simulink model "Multiplier"  (R2017b)
settings: Solver=ode45  StartTime=0.0  StopTime=10.0  RelTol=1e-3  EnableMultiTasking=on
libraries: hdlsllib x17
(part 2 of 3)

== system Multiplier/8-bit_Multiplier/Multiplier/Multiplier Building Block54 ==
  Cin : Inport
  X : Inport  Port=2
  Y : Inport  Port=3
  Sum in : Inport  Port=4
  AND : Logic  IconShape=distinctive  AllPortsSameDT=off  OutDataTypeStr=boolean
  Full Adder : Subsystem
  Sum Out : Outport
  C Out : Outport  Port=2
  wires:
  Cin/1 -> Full Adder/3(Z)
  Sum in/1 -> Full Adder/1(X)
  AND/1 -> Full Adder/2(Y)
  Full Adder/1(S) -> Sum Out/1
  Y/1 -> AND/2
  X/1 -> AND/1
  Full Adder/2(C) -> C Out/1

== system Multiplier/8-bit_Multiplier/Multiplier/Multiplier Building Block55 ==
  Cin : Inport
  X : Inport  Port=2
  Y : Inport  Port=3
  Sum in : Inport  Port=4
  AND : Logic  IconShape=distinctive  AllPortsSameDT=off  OutDataTypeStr=boolean
  Full Adder : Subsystem
  Sum Out : Outport
  C Out : Outport  Port=2
  wires:
  Cin/1 -> Full Adder/3(Z)
  Sum in/1 -> Full Adder/1(X)
  AND/1 -> Full Adder/2(Y)
  Full Adder/1(S) -> Sum Out/1
  Y/1 -> AND/2
  X/1 -> AND/1
  Full Adder/2(C) -> C Out/1

== system Multiplier/8-bit_Multiplier/Multiplier/Multiplier Building Block56 ==
  Cin : Inport
  X : Inport  Port=2
  Y : Inport  Port=3
  Sum in : Inport  Port=4
  AND : Logic  IconShape=distinctive  AllPortsSameDT=off  OutDataTypeStr=boolean
  Full Adder : Subsystem
  Sum Out : Outport
  C Out : Outport  Port=2
  wires:
  Cin/1 -> Full Adder/3(Z)
  Sum in/1 -> Full Adder/1(X)
  AND/1 -> Full Adder/2(Y)
  Full Adder/1(S) -> Sum Out/1
  Y/1 -> AND/2
  X/1 -> AND/1
  Full Adder/2(C) -> C Out/1

== system Multiplier/8-bit_Multiplier/Multiplier/Multiplier Building Block57 ==
  Cin : Inport
  X : Inport  Port=2
  Y : Inport  Port=3
  Sum in : Inport  Port=4
  AND : Logic  IconShape=distinctive  AllPortsSameDT=off  OutDataTypeStr=boolean
  Full Adder : Subsystem
  Sum Out : Outport
  C Out : Outport  Port=2
  wires:
  Cin/1 -> Full Adder/3(Z)
  Sum in/1 -> Full Adder/1(X)
  AND/1 -> Full Adder/2(Y)
  Full Adder/1(S) -> Sum Out/1
  Y/1 -> AND/2
  X/1 -> AND/1
  Full Adder/2(C) -> C Out/1

== system Multiplier/8-bit_Multiplier/Multiplier/Multiplier Building Block58 ==
  Cin : Inport
  X : Inport  Port=2
  Y : Inport  Port=3
  Sum in : Inport  Port=4
  AND : Logic  IconShape=distinctive  AllPortsSameDT=off  OutDataTypeStr=boolean
  Full Adder : Subsystem
  Sum Out : Outport
  C Out : Outport  Port=2
  wires:
  Cin/1 -> Full Adder/3(Z)
  Sum in/1 -> Full Adder/1(X)
  AND/1 -> Full Adder/2(Y)
  Full Adder/1(S) -> Sum Out/1
  Y/1 -> AND/2
  X/1 -> AND/1
  Full Adder/2(C) -> C Out/1

== system Multiplier/8-bit_Multiplier/Multiplier/Multiplier Building Block59 ==
  Cin : Inport
  X : Inport  Port=2
  Y : Inport  Port=3
  Sum in : Inport  Port=4
  AND : Logic  IconShape=distinctive  AllPortsSameDT=off  OutDataTypeStr=boolean
  Full Adder : Subsystem
  Sum Out : Outport
  C Out : Outport  Port=2
  wires:
  Cin/1 -> Full Adder/3(Z)
  Sum in/1 -> Full Adder/1(X)
  AND/1 -> Full Adder/2(Y)
  Full Adder/1(S) -> Sum Out/1
  Y/1 -> AND/2
  X/1 -> AND/1
  Full Adder/2(C) -> C Out/1

== system Multiplier/8-bit_Multiplier/Multiplier/Multiplier Building Block6 ==
  Cin : Inport
  X : Inport  Port=2
  Y : Inport  Port=3
  Sum in : Inport  Port=4
  AND : Logic  IconShape=distinctive  AllPortsSameDT=off  OutDataTypeStr=boolean
  Full Adder : Subsystem
  Sum Out : Outport
  C Out : Outport  Port=2
  wires:
  Cin/1 -> Full Adder/3(Z)
  Sum in/1 -> Full Adder/1(X)
  AND/1 -> Full Adder/2(Y)
  Full Adder/1(S) -> Sum Out/1
  Y/1 -> AND/2
  X/1 -> AND/1
  Full Adder/2(C) -> C Out/1

== system Multiplier/8-bit_Multiplier/Multiplier/Multiplier Building Block60 ==
  Cin : Inport
  X : Inport  Port=2
  Y : Inport  Port=3
  Sum in : Inport  Port=4
  AND : Logic  IconShape=distinctive  AllPortsSameDT=off  OutDataTypeStr=boolean
  Full Adder : Subsystem
  Sum Out : Outport
  C Out : Outport  Port=2
  wires:
  Cin/1 -> Full Adder/3(Z)
  Sum in/1 -> Full Adder/1(X)
  AND/1 -> Full Adder/2(Y)
  Full Adder/1(S) -> Sum Out/1
  Y/1 -> AND/2
  X/1 -> AND/1
  Full Adder/2(C) -> C Out/1

== system Multiplier/8-bit_Multiplier/Multiplier/Multiplier Building Block61 ==
  Cin : Inport
  X : Inport  Port=2
  Y : Inport  Port=3
  Sum in : Inport  Port=4
  AND : Logic  IconShape=distinctive  AllPortsSameDT=off  OutDataTypeStr=boolean
  Full Adder : Subsystem
  Sum Out : Outport
  C Out : Outport  Port=2
  wires:
  Cin/1 -> Full Adder/3(Z)
  Sum in/1 -> Full Adder/1(X)
  AND/1 -> Full Adder/2(Y)
  Full Adder/1(S) -> Sum Out/1
  Y/1 -> AND/2
  X/1 -> AND/1
  Full Adder/2(C) -> C Out/1

== system Multiplier/8-bit_Multiplier/Multiplier/Multiplier Building Block62 ==
  Cin : Inport
  X : Inport  Port=2
  Y : Inport  Port=3
  Sum in : Inport  Port=4
  AND : Logic  IconShape=distinctive  AllPortsSameDT=off  OutDataTypeStr=boolean
  Full Adder : Subsystem
  Sum Out : Outport
  C Out : Outport  Port=2
  wires:
  Cin/1 -> Full Adder/3(Z)
  Sum in/1 -> Full Adder/1(X)
  AND/1 -> Full Adder/2(Y)
  Full Adder/1(S) -> Sum Out/1
  Y/1 -> AND/2
  X/1 -> AND/1
  Full Adder/2(C) -> C Out/1

== system Multiplier/8-bit_Multiplier/Multiplier/Multiplier Building Block63 ==
  Cin : Inport
  X : Inport  Port=2
  Y : Inport  Port=3
  Sum in : Inport  Port=4
  AND : Logic  IconShape=distinctive  AllPortsSameDT=off  OutDataTypeStr=boolean
  Full Adder : Subsystem
  Sum Out : Outport
  C Out : Outport  Port=2
  wires:
  Cin/1 -> Full Adder/3(Z)
  Sum in/1 -> Full Adder/1(X)
  AND/1 -> Full Adder/2(Y)
  Full Adder/1(S) -> Sum Out/1
  Y/1 -> AND/2
  X/1 -> AND/1
  Full Adder/2(C) -> C Out/1

== system Multiplier/8-bit_Multiplier/Multiplier/Multiplier Building Block7 ==
  Cin : Inport
  X : Inport  Port=2
  Y : Inport  Port=3
  Sum in : Inport  Port=4
  AND : Logic  IconShape=distinctive  AllPortsSameDT=off  OutDataTypeStr=boolean
  Full Adder : Subsystem
  Sum Out : Outport
  C Out : Outport  Port=2
  wires:
  Cin/1 -> Full Adder/3(Z)
  Sum in/1 -> Full Adder/1(X)
  AND/1 -> Full Adder/2(Y)
  Full Adder/1(S) -> Sum Out/1
  Y/1 -> AND/2
  X/1 -> AND/1
  Full Adder/2(C) -> C Out/1

== system Multiplier/8-bit_Multiplier/Multiplier/Multiplier Building Block8 ==
  Cin : Inport
  X : Inport  Port=2
  Y : Inport  Port=3
  Sum in : Inport  Port=4
  AND : Logic  IconShape=distinctive  AllPortsSameDT=off  OutDataTypeStr=boolean
  Full Adder : Subsystem
  Sum Out : Outport
  C Out : Outport  Port=2
  wires:
  Cin/1 -> Full Adder/3(Z)
  Sum in/1 -> Full Adder/1(X)
  AND/1 -> Full Adder/2(Y)
  Full Adder/1(S) -> Sum Out/1
  Y/1 -> AND/2
  X/1 -> AND/1
  Full Adder/2(C) -> C Out/1

== system Multiplier/8-bit_Multiplier/Multiplier/Multiplier Building Block9 ==
  Cin : Inport
  X : Inport  Port=2
  Y : Inport  Port=3
  Sum in : Inport  Port=4
  AND : Logic  IconShape=distinctive  AllPortsSameDT=off  OutDataTypeStr=boolean
  Full Adder : Subsystem
  Sum Out : Outport
  C Out : Outport  Port=2
  wires:
  Cin/1 -> Full Adder/3(Z)
  Sum in/1 -> Full Adder/1(X)
  AND/1 -> Full Adder/2(Y)
  Full Adder/1(S) -> Sum Out/1
  Y/1 -> AND/2
  X/1 -> AND/1
  Full Adder/2(C) -> C Out/1

== system Multiplier/8-bit_Multiplier/Multiplier/Multiplier Building Block/Full Adder ==
  X : Inport
  Y : Inport  Port=2
  Z : Inport  Port=3
  Half Adder : Subsystem
  Half Adder1 : Subsystem
  OR : Logic  Operator=OR  IconShape=distinctive  AllPortsSameDT=off  OutDataTypeStr=boolean
  S : Outport
  C : Outport  Port=2
  wires:
  Half Adder1/1(Sum) -> S/1
  Half Adder/1(Sum) -> Half Adder1/1(A)
  Half Adder/2(Carry) -> OR/2
  X/1 -> Half Adder/1(A)
  Z/1 -> Half Adder1/2(B)
  OR/1 -> C/1
  Y/1 -> Half Adder/2(B)
  Half Adder1/2(Carry) -> OR/1

== system Multiplier/8-bit_Multiplier/Multiplier/Multiplier Building Block1/Full Adder ==
  X : Inport
  Y : Inport  Port=2
  Z : Inport  Port=3
  Half Adder : Subsystem
  Half Adder1 : Subsystem
  OR : Logic  Operator=OR  IconShape=distinctive  AllPortsSameDT=off  OutDataTypeStr=boolean
  S : Outport
  C : Outport  Port=2
  wires:
  Half Adder1/1(Sum) -> S/1
  Half Adder/1(Sum) -> Half Adder1/1(A)
  Half Adder/2(Carry) -> OR/2
  X/1 -> Half Adder/1(A)
  Z/1 -> Half Adder1/2(B)
  OR/1 -> C/1
  Y/1 -> Half Adder/2(B)
  Half Adder1/2(Carry) -> OR/1

== system Multiplier/8-bit_Multiplier/Multiplier/Multiplier Building Block10/Full Adder ==
  X : Inport
  Y : Inport  Port=2
  Z : Inport  Port=3
  Half Adder : Subsystem
  Half Adder1 : Subsystem
  OR : Logic  Operator=OR  IconShape=distinctive  AllPortsSameDT=off  OutDataTypeStr=boolean
  S : Outport
  C : Outport  Port=2
  wires:
  Half Adder1/1(Sum) -> S/1
  Half Adder/1(Sum) -> Half Adder1/1(A)
  Half Adder/2(Carry) -> OR/2
  X/1 -> Half Adder/1(A)
  Z/1 -> Half Adder1/2(B)
  OR/1 -> C/1
  Y/1 -> Half Adder/2(B)
  Half Adder1/2(Carry) -> OR/1

== system Multiplier/8-bit_Multiplier/Multiplier/Multiplier Building Block11/Full Adder ==
  X : Inport
  Y : Inport  Port=2
  Z : Inport  Port=3
  Half Adder : Subsystem
  Half Adder1 : Subsystem
  OR : Logic  Operator=OR  IconShape=distinctive  AllPortsSameDT=off  OutDataTypeStr=boolean
  S : Outport
  C : Outport  Port=2
  wires:
  Half Adder1/1(Sum) -> S/1
  Half Adder/1(Sum) -> Half Adder1/1(A)
  Half Adder/2(Carry) -> OR/2
  X/1 -> Half Adder/1(A)
  Z/1 -> Half Adder1/2(B)
  OR/1 -> C/1
  Y/1 -> Half Adder/2(B)
  Half Adder1/2(Carry) -> OR/1

== system Multiplier/8-bit_Multiplier/Multiplier/Multiplier Building Block12/Full Adder ==
  X : Inport
  Y : Inport  Port=2
  Z : Inport  Port=3
  Half Adder : Subsystem
  Half Adder1 : Subsystem
  OR : Logic  Operator=OR  IconShape=distinctive  AllPortsSameDT=off  OutDataTypeStr=boolean
  S : Outport
  C : Outport  Port=2
  wires:
  Half Adder1/1(Sum) -> S/1
  Half Adder/1(Sum) -> Half Adder1/1(A)
  Half Adder/2(Carry) -> OR/2
  X/1 -> Half Adder/1(A)
  Z/1 -> Half Adder1/2(B)
  OR/1 -> C/1
  Y/1 -> Half Adder/2(B)
  Half Adder1/2(Carry) -> OR/1

== system Multiplier/8-bit_Multiplier/Multiplier/Multiplier Building Block13/Full Adder ==
  X : Inport
  Y : Inport  Port=2
  Z : Inport  Port=3
  Half Adder : Subsystem
  Half Adder1 : Subsystem
  OR : Logic  Operator=OR  IconShape=distinctive  AllPortsSameDT=off  OutDataTypeStr=boolean
  S : Outport
  C : Outport  Port=2
  wires:
  Half Adder1/1(Sum) -> S/1
  Half Adder/1(Sum) -> Half Adder1/1(A)
  Half Adder/2(Carry) -> OR/2
  X/1 -> Half Adder/1(A)
  Z/1 -> Half Adder1/2(B)
  OR/1 -> C/1
  Y/1 -> Half Adder/2(B)
  Half Adder1/2(Carry) -> OR/1

== system Multiplier/8-bit_Multiplier/Multiplier/Multiplier Building Block14/Full Adder ==
  X : Inport
  Y : Inport  Port=2
  Z : Inport  Port=3
  Half Adder : Subsystem
  Half Adder1 : Subsystem
  OR : Logic  Operator=OR  IconShape=distinctive  AllPortsSameDT=off  OutDataTypeStr=boolean
  S : Outport
  C : Outport  Port=2
  wires:
  Half Adder1/1(Sum) -> S/1
  Half Adder/1(Sum) -> Half Adder1/1(A)
  Half Adder/2(Carry) -> OR/2
  X/1 -> Half Adder/1(A)
  Z/1 -> Half Adder1/2(B)
  OR/1 -> C/1
  Y/1 -> Half Adder/2(B)
  Half Adder1/2(Carry) -> OR/1

== system Multiplier/8-bit_Multiplier/Multiplier/Multiplier Building Block15/Full Adder ==
  X : Inport
  Y : Inport  Port=2
  Z : Inport  Port=3
  Half Adder : Subsystem
  Half Adder1 : Subsystem
  OR : Logic  Operator=OR  IconShape=distinctive  AllPortsSameDT=off  OutDataTypeStr=boolean
  S : Outport
  C : Outport  Port=2
  wires:
  Half Adder1/1(Sum) -> S/1
  Half Adder/1(Sum) -> Half Adder1/1(A)
  Half Adder/2(Carry) -> OR/2
  X/1 -> Half Adder/1(A)
  Z/1 -> Half Adder1/2(B)
  OR/1 -> C/1
  Y/1 -> Half Adder/2(B)
  Half Adder1/2(Carry) -> OR/1

== system Multiplier/8-bit_Multiplier/Multiplier/Multiplier Building Block16/Full Adder ==
  X : Inport
  Y : Inport  Port=2
  Z : Inport  Port=3
  Half Adder : Subsystem
  Half Adder1 : Subsystem
  OR : Logic  Operator=OR  IconShape=distinctive  AllPortsSameDT=off  OutDataTypeStr=boolean
  S : Outport
  C : Outport  Port=2
  wires:
  Half Adder1/1(Sum) -> S/1
  Half Adder/1(Sum) -> Half Adder1/1(A)
  Half Adder/2(Carry) -> OR/2
  X/1 -> Half Adder/1(A)
  Z/1 -> Half Adder1/2(B)
  OR/1 -> C/1
  Y/1 -> Half Adder/2(B)
  Half Adder1/2(Carry) -> OR/1

== system Multiplier/8-bit_Multiplier/Multiplier/Multiplier Building Block17/Full Adder ==
  X : Inport
  Y : Inport  Port=2
  Z : Inport  Port=3
  Half Adder : Subsystem
  Half Adder1 : Subsystem
  OR : Logic  Operator=OR  IconShape=distinctive  AllPortsSameDT=off  OutDataTypeStr=boolean
  S : Outport
  C : Outport  Port=2
  wires:
  Half Adder1/1(Sum) -> S/1
  Half Adder/1(Sum) -> Half Adder1/1(A)
  Half Adder/2(Carry) -> OR/2
  X/1 -> Half Adder/1(A)
  Z/1 -> Half Adder1/2(B)
  OR/1 -> C/1
  Y/1 -> Half Adder/2(B)
  Half Adder1/2(Carry) -> OR/1

== system Multiplier/8-bit_Multiplier/Multiplier/Multiplier Building Block18/Full Adder ==
  X : Inport
  Y : Inport  Port=2
  Z : Inport  Port=3
  Half Adder : Subsystem
  Half Adder1 : Subsystem
  OR : Logic  Operator=OR  IconShape=distinctive  AllPortsSameDT=off  OutDataTypeStr=boolean
  S : Outport
  C : Outport  Port=2
  wires:
  Half Adder1/1(Sum) -> S/1
  Half Adder/1(Sum) -> Half Adder1/1(A)
  Half Adder/2(Carry) -> OR/2
  X/1 -> Half Adder/1(A)
  Z/1 -> Half Adder1/2(B)
  OR/1 -> C/1
  Y/1 -> Half Adder/2(B)
  Half Adder1/2(Carry) -> OR/1

== system Multiplier/8-bit_Multiplier/Multiplier/Multiplier Building Block19/Full Adder ==
  X : Inport
  Y : Inport  Port=2
  Z : Inport  Port=3
  Half Adder : Subsystem
  Half Adder1 : Subsystem
  OR : Logic  Operator=OR  IconShape=distinctive  AllPortsSameDT=off  OutDataTypeStr=boolean
  S : Outport
  C : Outport  Port=2
  wires:
  Half Adder1/1(Sum) -> S/1
  Half Adder/1(Sum) -> Half Adder1/1(A)
  Half Adder/2(Carry) -> OR/2
  X/1 -> Half Adder/1(A)
  Z/1 -> Half Adder1/2(B)
  OR/1 -> C/1
  Y/1 -> Half Adder/2(B)
  Half Adder1/2(Carry) -> OR/1

== system Multiplier/8-bit_Multiplier/Multiplier/Multiplier Building Block2/Full Adder ==
  X : Inport
  Y : Inport  Port=2
  Z : Inport  Port=3
  Half Adder : Subsystem
  Half Adder1 : Subsystem
  OR : Logic  Operator=OR  IconShape=distinctive  AllPortsSameDT=off  OutDataTypeStr=boolean
  S : Outport
  C : Outport  Port=2
  wires:
  Half Adder1/1(Sum) -> S/1
  Half Adder/1(Sum) -> Half Adder1/1(A)
  Half Adder/2(Carry) -> OR/2
  X/1 -> Half Adder/1(A)
  Z/1 -> Half Adder1/2(B)
  OR/1 -> C/1
  Y/1 -> Half Adder/2(B)
  Half Adder1/2(Carry) -> OR/1

== system Multiplier/8-bit_Multiplier/Multiplier/Multiplier Building Block20/Full Adder ==
  X : Inport
  Y : Inport  Port=2
  Z : Inport  Port=3
  Half Adder : Subsystem
  Half Adder1 : Subsystem
  OR : Logic  Operator=OR  IconShape=distinctive  AllPortsSameDT=off  OutDataTypeStr=boolean
  S : Outport
  C : Outport  Port=2
  wires:
  Half Adder1/1(Sum) -> S/1
  Half Adder/1(Sum) -> Half Adder1/1(A)
  Half Adder/2(Carry) -> OR/2
  X/1 -> Half Adder/1(A)
  Z/1 -> Half Adder1/2(B)
  OR/1 -> C/1
  Y/1 -> Half Adder/2(B)
  Half Adder1/2(Carry) -> OR/1

== system Multiplier/8-bit_Multiplier/Multiplier/Multiplier Building Block21/Full Adder ==
  X : Inport
  Y : Inport  Port=2
  Z : Inport  Port=3
  Half Adder : Subsystem
  Half Adder1 : Subsystem
  OR : Logic  Operator=OR  IconShape=distinctive  AllPortsSameDT=off  OutDataTypeStr=boolean
  S : Outport
  C : Outport  Port=2
  wires:
  Half Adder1/1(Sum) -> S/1
  Half Adder/1(Sum) -> Half Adder1/1(A)
  Half Adder/2(Carry) -> OR/2
  X/1 -> Half Adder/1(A)
  Z/1 -> Half Adder1/2(B)
  OR/1 -> C/1
  Y/1 -> Half Adder/2(B)
  Half Adder1/2(Carry) -> OR/1

== system Multiplier/8-bit_Multiplier/Multiplier/Multiplier Building Block22/Full Adder ==
  X : Inport
  Y : Inport  Port=2
  Z : Inport  Port=3
  Half Adder : Subsystem
  Half Adder1 : Subsystem
  OR : Logic  Operator=OR  IconShape=distinctive  AllPortsSameDT=off  OutDataTypeStr=boolean
  S : Outport
  C : Outport  Port=2
  wires:
  Half Adder1/1(Sum) -> S/1
  Half Adder/1(Sum) -> Half Adder1/1(A)
  Half Adder/2(Carry) -> OR/2
  X/1 -> Half Adder/1(A)
  Z/1 -> Half Adder1/2(B)
  OR/1 -> C/1
  Y/1 -> Half Adder/2(B)
  Half Adder1/2(Carry) -> OR/1

== system Multiplier/8-bit_Multiplier/Multiplier/Multiplier Building Block23/Full Adder ==
  X : Inport
  Y : Inport  Port=2
  Z : Inport  Port=3
  Half Adder : Subsystem
  Half Adder1 : Subsystem
  OR : Logic  Operator=OR  IconShape=distinctive  AllPortsSameDT=off  OutDataTypeStr=boolean
  S : Outport
  C : Outport  Port=2
  wires:
  Half Adder1/1(Sum) -> S/1
  Half Adder/1(Sum) -> Half Adder1/1(A)
  Half Adder/2(Carry) -> OR/2
  X/1 -> Half Adder/1(A)
  Z/1 -> Half Adder1/2(B)
  OR/1 -> C/1
  Y/1 -> Half Adder/2(B)
  Half Adder1/2(Carry) -> OR/1

== system Multiplier/8-bit_Multiplier/Multiplier/Multiplier Building Block24/Full Adder ==
  X : Inport
  Y : Inport  Port=2
  Z : Inport  Port=3
  Half Adder : Subsystem
  Half Adder1 : Subsystem
  OR : Logic  Operator=OR  IconShape=distinctive  AllPortsSameDT=off  OutDataTypeStr=boolean
  S : Outport
  C : Outport  Port=2
  wires:
  Half Adder1/1(Sum) -> S/1
  Half Adder/1(Sum) -> Half Adder1/1(A)
  Half Adder/2(Carry) -> OR/2
  X/1 -> Half Adder/1(A)
  Z/1 -> Half Adder1/2(B)
  OR/1 -> C/1
  Y/1 -> Half Adder/2(B)
  Half Adder1/2(Carry) -> OR/1

== system Multiplier/8-bit_Multiplier/Multiplier/Multiplier Building Block25/Full Adder ==
  X : Inport
  Y : Inport  Port=2
  Z : Inport  Port=3
  Half Adder : Subsystem
  Half Adder1 : Subsystem
  OR : Logic  Operator=OR  IconShape=distinctive  AllPortsSameDT=off  OutDataTypeStr=boolean
  S : Outport
  C : Outport  Port=2
  wires:
  Half Adder1/1(Sum) -> S/1
  Half Adder/1(Sum) -> Half Adder1/1(A)
  Half Adder/2(Carry) -> OR/2
  X/1 -> Half Adder/1(A)
  Z/1 -> Half Adder1/2(B)
  OR/1 -> C/1
  Y/1 -> Half Adder/2(B)
  Half Adder1/2(Carry) -> OR/1

== system Multiplier/8-bit_Multiplier/Multiplier/Multiplier Building Block26/Full Adder ==
  X : Inport
  Y : Inport  Port=2
  Z : Inport  Port=3
  Half Adder : Subsystem
  Half Adder1 : Subsystem
  OR : Logic  Operator=OR  IconShape=distinctive  AllPortsSameDT=off  OutDataTypeStr=boolean
  S : Outport
  C : Outport  Port=2
  wires:
  Half Adder1/1(Sum) -> S/1
  Half Adder/1(Sum) -> Half Adder1/1(A)
  Half Adder/2(Carry) -> OR/2
  X/1 -> Half Adder/1(A)
  Z/1 -> Half Adder1/2(B)
  OR/1 -> C/1
  Y/1 -> Half Adder/2(B)
  Half Adder1/2(Carry) -> OR/1

== system Multiplier/8-bit_Multiplier/Multiplier/Multiplier Building Block27/Full Adder ==
  X : Inport
  Y : Inport  Port=2
  Z : Inport  Port=3
  Half Adder : Subsystem
  Half Adder1 : Subsystem
  OR : Logic  Operator=OR  IconShape=distinctive  AllPortsSameDT=off  OutDataTypeStr=boolean
  S : Outport
  C : Outport  Port=2
  wires:
  Half Adder1/1(Sum) -> S/1
  Half Adder/1(Sum) -> Half Adder1/1(A)
  Half Adder/2(Carry) -> OR/2
  X/1 -> Half Adder/1(A)
  Z/1 -> Half Adder1/2(B)
  OR/1 -> C/1
  Y/1 -> Half Adder/2(B)
  Half Adder1/2(Carry) -> OR/1

== system Multiplier/8-bit_Multiplier/Multiplier/Multiplier Building Block28/Full Adder ==
  X : Inport
  Y : Inport  Port=2
  Z : Inport  Port=3
  Half Adder : Subsystem
  Half Adder1 : Subsystem
  OR : Logic  Operator=OR  IconShape=distinctive  AllPortsSameDT=off  OutDataTypeStr=boolean
  S : Outport
  C : Outport  Port=2
  wires:
  Half Adder1/1(Sum) -> S/1
  Half Adder/1(Sum) -> Half Adder1/1(A)
  Half Adder/2(Carry) -> OR/2
  X/1 -> Half Adder/1(A)
  Z/1 -> Half Adder1/2(B)
  OR/1 -> C/1
  Y/1 -> Half Adder/2(B)
  Half Adder1/2(Carry) -> OR/1

== system Multiplier/8-bit_Multiplier/Multiplier/Multiplier Building Block29/Full Adder ==
  X : Inport
  Y : Inport  Port=2
  Z : Inport  Port=3
  Half Adder : Subsystem
  Half Adder1 : Subsystem
  OR : Logic  Operator=OR  IconShape=distinctive  AllPortsSameDT=off  OutDataTypeStr=boolean
  S : Outport
  C : Outport  Port=2
  wires:
  Half Adder1/1(Sum) -> S/1
  Half Adder/1(Sum) -> Half Adder1/1(A)
  Half Adder/2(Carry) -> OR/2
  X/1 -> Half Adder/1(A)
  Z/1 -> Half Adder1/2(B)
  OR/1 -> C/1
  Y/1 -> Half Adder/2(B)
  Half Adder1/2(Carry) -> OR/1

== system Multiplier/8-bit_Multiplier/Multiplier/Multiplier Building Block3/Full Adder ==
  X : Inport
  Y : Inport  Port=2
  Z : Inport  Port=3
  Half Adder : Subsystem
  Half Adder1 : Subsystem
  OR : Logic  Operator=OR  IconShape=distinctive  AllPortsSameDT=off  OutDataTypeStr=boolean
  S : Outport
  C : Outport  Port=2
  wires:
  Half Adder1/1(Sum) -> S/1
  Half Adder/1(Sum) -> Half Adder1/1(A)
  Half Adder/2(Carry) -> OR/2
  X/1 -> Half Adder/1(A)
  Z/1 -> Half Adder1/2(B)
  OR/1 -> C/1
  Y/1 -> Half Adder/2(B)
  Half Adder1/2(Carry) -> OR/1

== system Multiplier/8-bit_Multiplier/Multiplier/Multiplier Building Block30/Full Adder ==
  X : Inport
  Y : Inport  Port=2
  Z : Inport  Port=3
  Half Adder : Subsystem
  Half Adder1 : Subsystem
  OR : Logic  Operator=OR  IconShape=distinctive  AllPortsSameDT=off  OutDataTypeStr=boolean
  S : Outport
  C : Outport  Port=2
  wires:
  Half Adder1/1(Sum) -> S/1
  Half Adder/1(Sum) -> Half Adder1/1(A)
  Half Adder/2(Carry) -> OR/2
  X/1 -> Half Adder/1(A)
  Z/1 -> Half Adder1/2(B)
  OR/1 -> C/1
  Y/1 -> Half Adder/2(B)
  Half Adder1/2(Carry) -> OR/1

== system Multiplier/8-bit_Multiplier/Multiplier/Multiplier Building Block31/Full Adder ==
  X : Inport
  Y : Inport  Port=2
  Z : Inport  Port=3
  Half Adder : Subsystem
  Half Adder1 : Subsystem
  OR : Logic  Operator=OR  IconShape=distinctive  AllPortsSameDT=off  OutDataTypeStr=boolean
  S : Outport
  C : Outport  Port=2
  wires:
  Half Adder1/1(Sum) -> S/1
  Half Adder/1(Sum) -> Half Adder1/1(A)
  Half Adder/2(Carry) -> OR/2
  X/1 -> Half Adder/1(A)
  Z/1 -> Half Adder1/2(B)
  OR/1 -> C/1
  Y/1 -> Half Adder/2(B)
  Half Adder1/2(Carry) -> OR/1

== system Multiplier/8-bit_Multiplier/Multiplier/Multiplier Building Block32/Full Adder ==
  X : Inport
  Y : Inport  Port=2
  Z : Inport  Port=3
  Half Adder : Subsystem
  Half Adder1 : Subsystem
  OR : Logic  Operator=OR  IconShape=distinctive  AllPortsSameDT=off  OutDataTypeStr=boolean
  S : Outport
  C : Outport  Port=2
  wires:
  Half Adder1/1(Sum) -> S/1
  Half Adder/1(Sum) -> Half Adder1/1(A)
  Half Adder/2(Carry) -> OR/2
  X/1 -> Half Adder/1(A)
  Z/1 -> Half Adder1/2(B)
  OR/1 -> C/1
  Y/1 -> Half Adder/2(B)
  Half Adder1/2(Carry) -> OR/1

== system Multiplier/8-bit_Multiplier/Multiplier/Multiplier Building Block33/Full Adder ==
  X : Inport
  Y : Inport  Port=2
  Z : Inport  Port=3
  Half Adder : Subsystem
  Half Adder1 : Subsystem
  OR : Logic  Operator=OR  IconShape=distinctive  AllPortsSameDT=off  OutDataTypeStr=boolean
  S : Outport
  C : Outport  Port=2
  wires:
  Half Adder1/1(Sum) -> S/1
  Half Adder/1(Sum) -> Half Adder1/1(A)
  Half Adder/2(Carry) -> OR/2
  X/1 -> Half Adder/1(A)
  Z/1 -> Half Adder1/2(B)
  OR/1 -> C/1
  Y/1 -> Half Adder/2(B)
  Half Adder1/2(Carry) -> OR/1

== system Multiplier/8-bit_Multiplier/Multiplier/Multiplier Building Block34/Full Adder ==
  X : Inport
  Y : Inport  Port=2
  Z : Inport  Port=3
  Half Adder : Subsystem
  Half Adder1 : Subsystem
  OR : Logic  Operator=OR  IconShape=distinctive  AllPortsSameDT=off  OutDataTypeStr=boolean
  S : Outport
  C : Outport  Port=2
  wires:
  Half Adder1/1(Sum) -> S/1
  Half Adder/1(Sum) -> Half Adder1/1(A)
  Half Adder/2(Carry) -> OR/2
  X/1 -> Half Adder/1(A)
  Z/1 -> Half Adder1/2(B)
  OR/1 -> C/1
  Y/1 -> Half Adder/2(B)
  Half Adder1/2(Carry) -> OR/1

== system Multiplier/8-bit_Multiplier/Multiplier/Multiplier Building Block35/Full Adder ==
  X : Inport
  Y : Inport  Port=2
  Z : Inport  Port=3
  Half Adder : Subsystem
  Half Adder1 : Subsystem
  OR : Logic  Operator=OR  IconShape=distinctive  AllPortsSameDT=off  OutDataTypeStr=boolean
  S : Outport
  C : Outport  Port=2
  wires:
  Half Adder1/1(Sum) -> S/1
  Half Adder/1(Sum) -> Half Adder1/1(A)
  Half Adder/2(Carry) -> OR/2
  X/1 -> Half Adder/1(A)
  Z/1 -> Half Adder1/2(B)
  OR/1 -> C/1
  Y/1 -> Half Adder/2(B)
  Half Adder1/2(Carry) -> OR/1

== system Multiplier/8-bit_Multiplier/Multiplier/Multiplier Building Block36/Full Adder ==
  X : Inport
  Y : Inport  Port=2
  Z : Inport  Port=3
  Half Adder : Subsystem
  Half Adder1 : Subsystem
  OR : Logic  Operator=OR  IconShape=distinctive  AllPortsSameDT=off  OutDataTypeStr=boolean
  S : Outport
  C : Outport  Port=2
  wires:
  Half Adder1/1(Sum) -> S/1
  Half Adder/1(Sum) -> Half Adder1/1(A)
  Half Adder/2(Carry) -> OR/2
  X/1 -> Half Adder/1(A)
  Z/1 -> Half Adder1/2(B)
  OR/1 -> C/1
  Y/1 -> Half Adder/2(B)
  Half Adder1/2(Carry) -> OR/1

== system Multiplier/8-bit_Multiplier/Multiplier/Multiplier Building Block37/Full Adder ==
  X : Inport
  Y : Inport  Port=2
  Z : Inport  Port=3
  Half Adder : Subsystem
  Half Adder1 : Subsystem
  OR : Logic  Operator=OR  IconShape=distinctive  AllPortsSameDT=off  OutDataTypeStr=boolean
  S : Outport
  C : Outport  Port=2
  wires:
  Half Adder1/1(Sum) -> S/1
  Half Adder/1(Sum) -> Half Adder1/1(A)
  Half Adder/2(Carry) -> OR/2
  X/1 -> Half Adder/1(A)
  Z/1 -> Half Adder1/2(B)
  OR/1 -> C/1
  Y/1 -> Half Adder/2(B)
  Half Adder1/2(Carry) -> OR/1

== system Multiplier/8-bit_Multiplier/Multiplier/Multiplier Building Block38/Full Adder ==
  X : Inport
  Y : Inport  Port=2
  Z : Inport  Port=3
  Half Adder : Subsystem
  Half Adder1 : Subsystem
  OR : Logic  Operator=OR  IconShape=distinctive  AllPortsSameDT=off  OutDataTypeStr=boolean
  S : Outport
  C : Outport  Port=2
  wires:
  Half Adder1/1(Sum) -> S/1
  Half Adder/1(Sum) -> Half Adder1/1(A)
  Half Adder/2(Carry) -> OR/2
  X/1 -> Half Adder/1(A)
  Z/1 -> Half Adder1/2(B)
  OR/1 -> C/1
  Y/1 -> Half Adder/2(B)
  Half Adder1/2(Carry) -> OR/1

== system Multiplier/8-bit_Multiplier/Multiplier/Multiplier Building Block39/Full Adder ==
  X : Inport
  Y : Inport  Port=2
  Z : Inport  Port=3
  Half Adder : Subsystem
  Half Adder1 : Subsystem
  OR : Logic  Operator=OR  IconShape=distinctive  AllPortsSameDT=off  OutDataTypeStr=boolean
  S : Outport
  C : Outport  Port=2
  wires:
  Half Adder1/1(Sum) -> S/1
  Half Adder/1(Sum) -> Half Adder1/1(A)
  Half Adder/2(Carry) -> OR/2
  X/1 -> Half Adder/1(A)
  Z/1 -> Half Adder1/2(B)
  OR/1 -> C/1
  Y/1 -> Half Adder/2(B)
  Half Adder1/2(Carry) -> OR/1

== system Multiplier/8-bit_Multiplier/Multiplier/Multiplier Building Block4/Full Adder ==
  X : Inport
  Y : Inport  Port=2
  Z : Inport  Port=3
  Half Adder : Subsystem
  Half Adder1 : Subsystem
  OR : Logic  Operator=OR  IconShape=distinctive  AllPortsSameDT=off  OutDataTypeStr=boolean
  S : Outport
  C : Outport  Port=2
  wires:
  Half Adder1/1(Sum) -> S/1
  Half Adder/1(Sum) -> Half Adder1/1(A)
  Half Adder/2(Carry) -> OR/2
  X/1 -> Half Adder/1(A)
  Z/1 -> Half Adder1/2(B)
  OR/1 -> C/1
  Y/1 -> Half Adder/2(B)
  Half Adder1/2(Carry) -> OR/1

== system Multiplier/8-bit_Multiplier/Multiplier/Multiplier Building Block40/Full Adder ==
  X : Inport
  Y : Inport  Port=2
  Z : Inport  Port=3
  Half Adder : Subsystem
  Half Adder1 : Subsystem
  OR : Logic  Operator=OR  IconShape=distinctive  AllPortsSameDT=off  OutDataTypeStr=boolean
  S : Outport
  C : Outport  Port=2
  wires:
  Half Adder1/1(Sum) -> S/1
  Half Adder/1(Sum) -> Half Adder1/1(A)
  Half Adder/2(Carry) -> OR/2
  X/1 -> Half Adder/1(A)
  Z/1 -> Half Adder1/2(B)
  OR/1 -> C/1
  Y/1 -> Half Adder/2(B)
  Half Adder1/2(Carry) -> OR/1

== system Multiplier/8-bit_Multiplier/Multiplier/Multiplier Building Block41/Full Adder ==
  X : Inport
  Y : Inport  Port=2
  Z : Inport  Port=3
  Half Adder : Subsystem
  Half Adder1 : Subsystem
  OR : Logic  Operator=OR  IconShape=distinctive  AllPortsSameDT=off  OutDataTypeStr=boolean
  S : Outport
  C : Outport  Port=2
  wires:
  Half Adder1/1(Sum) -> S/1
  Half Adder/1(Sum) -> Half Adder1/1(A)
  Half Adder/2(Carry) -> OR/2
  X/1 -> Half Adder/1(A)
  Z/1 -> Half Adder1/2(B)
  OR/1 -> C/1
  Y/1 -> Half Adder/2(B)
  Half Adder1/2(Carry) -> OR/1

== system Multiplier/8-bit_Multiplier/Multiplier/Multiplier Building Block42/Full Adder ==
  X : Inport
  Y : Inport  Port=2
  Z : Inport  Port=3
  Half Adder : Subsystem
  Half Adder1 : Subsystem
  OR : Logic  Operator=OR  IconShape=distinctive  AllPortsSameDT=off  OutDataTypeStr=boolean
  S : Outport
  C : Outport  Port=2
  wires:
  Half Adder1/1(Sum) -> S/1
  Half Adder/1(Sum) -> Half Adder1/1(A)
  Half Adder/2(Carry) -> OR/2
  X/1 -> Half Adder/1(A)
  Z/1 -> Half Adder1/2(B)
  OR/1 -> C/1
  Y/1 -> Half Adder/2(B)
  Half Adder1/2(Carry) -> OR/1

== system Multiplier/8-bit_Multiplier/Multiplier/Multiplier Building Block43/Full Adder ==
  X : Inport
  Y : Inport  Port=2
  Z : Inport  Port=3
  Half Adder : Subsystem
  Half Adder1 : Subsystem
  OR : Logic  Operator=OR  IconShape=distinctive  AllPortsSameDT=off  OutDataTypeStr=boolean
  S : Outport
  C : Outport  Port=2
  wires:
  Half Adder1/1(Sum) -> S/1
  Half Adder/1(Sum) -> Half Adder1/1(A)
  Half Adder/2(Carry) -> OR/2
  X/1 -> Half Adder/1(A)
  Z/1 -> Half Adder1/2(B)
  OR/1 -> C/1
  Y/1 -> Half Adder/2(B)
  Half Adder1/2(Carry) -> OR/1

== system Multiplier/8-bit_Multiplier/Multiplier/Multiplier Building Block44/Full Adder ==
  X : Inport
  Y : Inport  Port=2
  Z : Inport  Port=3
  Half Adder : Subsystem
  Half Adder1 : Subsystem
  OR : Logic  Operator=OR  IconShape=distinctive  AllPortsSameDT=off  OutDataTypeStr=boolean
  S : Outport
  C : Outport  Port=2
  wires:
  Half Adder1/1(Sum) -> S/1
  Half Adder/1(Sum) -> Half Adder1/1(A)
  Half Adder/2(Carry) -> OR/2
  X/1 -> Half Adder/1(A)
  Z/1 -> Half Adder1/2(B)
  OR/1 -> C/1
  Y/1 -> Half Adder/2(B)
  Half Adder1/2(Carry) -> OR/1

== system Multiplier/8-bit_Multiplier/Multiplier/Multiplier Building Block45/Full Adder ==
  X : Inport
  Y : Inport  Port=2
  Z : Inport  Port=3
  Half Adder : Subsystem
  Half Adder1 : Subsystem
  OR : Logic  Operator=OR  IconShape=distinctive  AllPortsSameDT=off  OutDataTypeStr=boolean
  S : Outport
  C : Outport  Port=2
  wires:
  Half Adder1/1(Sum) -> S/1
  Half Adder/1(Sum) -> Half Adder1/1(A)
  Half Adder/2(Carry) -> OR/2
  X/1 -> Half Adder/1(A)
  Z/1 -> Half Adder1/2(B)
  OR/1 -> C/1
  Y/1 -> Half Adder/2(B)
  Half Adder1/2(Carry) -> OR/1

== system Multiplier/8-bit_Multiplier/Multiplier/Multiplier Building Block46/Full Adder ==
  X : Inport
  Y : Inport  Port=2
  Z : Inport  Port=3
  Half Adder : Subsystem
  Half Adder1 : Subsystem
  OR : Logic  Operator=OR  IconShape=distinctive  AllPortsSameDT=off  OutDataTypeStr=boolean
  S : Outport
  C : Outport  Port=2
  wires:
  Half Adder1/1(Sum) -> S/1
  Half Adder/1(Sum) -> Half Adder1/1(A)
  Half Adder/2(Carry) -> OR/2
  X/1 -> Half Adder/1(A)
  Z/1 -> Half Adder1/2(B)
  OR/1 -> C/1
  Y/1 -> Half Adder/2(B)
  Half Adder1/2(Carry) -> OR/1

== system Multiplier/8-bit_Multiplier/Multiplier/Multiplier Building Block47/Full Adder ==
  X : Inport
  Y : Inport  Port=2
  Z : Inport  Port=3
  Half Adder : Subsystem
  Half Adder1 : Subsystem
  OR : Logic  Operator=OR  IconShape=distinctive  AllPortsSameDT=off  OutDataTypeStr=boolean
  S : Outport
  C : Outport  Port=2
  wires:
  Half Adder1/1(Sum) -> S/1
  Half Adder/1(Sum) -> Half Adder1/1(A)
  Half Adder/2(Carry) -> OR/2
  X/1 -> Half Adder/1(A)
  Z/1 -> Half Adder1/2(B)
  OR/1 -> C/1
  Y/1 -> Half Adder/2(B)
  Half Adder1/2(Carry) -> OR/1

== system Multiplier/8-bit_Multiplier/Multiplier/Multiplier Building Block48/Full Adder ==
  X : Inport
  Y : Inport  Port=2
  Z : Inport  Port=3
  Half Adder : Subsystem
  Half Adder1 : Subsystem
  OR : Logic  Operator=OR  IconShape=distinctive  AllPortsSameDT=off  OutDataTypeStr=boolean
  S : Outport
  C : Outport  Port=2
  wires:
  Half Adder1/1(Sum) -> S/1
  Half Adder/1(Sum) -> Half Adder1/1(A)
  Half Adder/2(Carry) -> OR/2
  X/1 -> Half Adder/1(A)
  Z/1 -> Half Adder1/2(B)
  OR/1 -> C/1
  Y/1 -> Half Adder/2(B)
  Half Adder1/2(Carry) -> OR/1

== system Multiplier/8-bit_Multiplier/Multiplier/Multiplier Building Block49/Full Adder ==
  X : Inport
  Y : Inport  Port=2
  Z : Inport  Port=3
  Half Adder : Subsystem
  Half Adder1 : Subsystem
  OR : Logic  Operator=OR  IconShape=distinctive  AllPortsSameDT=off  OutDataTypeStr=boolean
  S : Outport
  C : Outport  Port=2
  wires:
  Half Adder1/1(Sum) -> S/1
  Half Adder/1(Sum) -> Half Adder1/1(A)
  Half Adder/2(Carry) -> OR/2
  X/1 -> Half Adder/1(A)
  Z/1 -> Half Adder1/2(B)
  OR/1 -> C/1
  Y/1 -> Half Adder/2(B)
  Half Adder1/2(Carry) -> OR/1

== system Multiplier/8-bit_Multiplier/Multiplier/Multiplier Building Block5/Full Adder ==
  X : Inport
  Y : Inport  Port=2
  Z : Inport  Port=3
  Half Adder : Subsystem
  Half Adder1 : Subsystem
  OR : Logic  Operator=OR  IconShape=distinctive  AllPortsSameDT=off  OutDataTypeStr=boolean
  S : Outport
  C : Outport  Port=2
  wires:
  Half Adder1/1(Sum) -> S/1
  Half Adder/1(Sum) -> Half Adder1/1(A)
  Half Adder/2(Carry) -> OR/2
  X/1 -> Half Adder/1(A)
  Z/1 -> Half Adder1/2(B)
  OR/1 -> C/1
  Y/1 -> Half Adder/2(B)
  Half Adder1/2(Carry) -> OR/1

== system Multiplier/8-bit_Multiplier/Multiplier/Multiplier Building Block50/Full Adder ==
  X : Inport
  Y : Inport  Port=2
  Z : Inport  Port=3
  Half Adder : Subsystem
  Half Adder1 : Subsystem
  OR : Logic  Operator=OR  IconShape=distinctive  AllPortsSameDT=off  OutDataTypeStr=boolean
  S : Outport
  C : Outport  Port=2
  wires:
  Half Adder1/1(Sum) -> S/1
  Half Adder/1(Sum) -> Half Adder1/1(A)
  Half Adder/2(Carry) -> OR/2
  X/1 -> Half Adder/1(A)
  Z/1 -> Half Adder1/2(B)
  OR/1 -> C/1
  Y/1 -> Half Adder/2(B)
  Half Adder1/2(Carry) -> OR/1

== system Multiplier/8-bit_Multiplier/Multiplier/Multiplier Building Block51/Full Adder ==
  X : Inport
  Y : Inport  Port=2
  Z : Inport  Port=3
  Half Adder : Subsystem
  Half Adder1 : Subsystem
  OR : Logic  Operator=OR  IconShape=distinctive  AllPortsSameDT=off  OutDataTypeStr=boolean
  S : Outport
  C : Outport  Port=2
  wires:
  Half Adder1/1(Sum) -> S/1
  Half Adder/1(Sum) -> Half Adder1/1(A)
  Half Adder/2(Carry) -> OR/2
  X/1 -> Half Adder/1(A)
  Z/1 -> Half Adder1/2(B)
  OR/1 -> C/1
  Y/1 -> Half Adder/2(B)
  Half Adder1/2(Carry) -> OR/1

== system Multiplier/8-bit_Multiplier/Multiplier/Multiplier Building Block52/Full Adder ==
  X : Inport
  Y : Inport  Port=2
  Z : Inport  Port=3
  Half Adder : Subsystem
  Half Adder1 : Subsystem
  OR : Logic  Operator=OR  IconShape=distinctive  AllPortsSameDT=off  OutDataTypeStr=boolean
  S : Outport
  C : Outport  Port=2
  wires:
  Half Adder1/1(Sum) -> S/1
  Half Adder/1(Sum) -> Half Adder1/1(A)
  Half Adder/2(Carry) -> OR/2
  X/1 -> Half Adder/1(A)
  Z/1 -> Half Adder1/2(B)
  OR/1 -> C/1
  Y/1 -> Half Adder/2(B)
  Half Adder1/2(Carry) -> OR/1

== system Multiplier/8-bit_Multiplier/Multiplier/Multiplier Building Block53/Full Adder ==
  X : Inport
  Y : Inport  Port=2
  Z : Inport  Port=3
  Half Adder : Subsystem
  Half Adder1 : Subsystem
  OR : Logic  Operator=OR  IconShape=distinctive  AllPortsSameDT=off  OutDataTypeStr=boolean
  S : Outport
  C : Outport  Port=2
  wires:
  Half Adder1/1(Sum) -> S/1
  Half Adder/1(Sum) -> Half Adder1/1(A)
  Half Adder/2(Carry) -> OR/2
  X/1 -> Half Adder/1(A)
  Z/1 -> Half Adder1/2(B)
  OR/1 -> C/1
  Y/1 -> Half Adder/2(B)
  Half Adder1/2(Carry) -> OR/1

== system Multiplier/8-bit_Multiplier/Multiplier/Multiplier Building Block54/Full Adder ==
  X : Inport
  Y : Inport  Port=2
  Z : Inport  Port=3
  Half Adder : Subsystem
  Half Adder1 : Subsystem
  OR : Logic  Operator=OR  IconShape=distinctive  AllPortsSameDT=off  OutDataTypeStr=boolean
  S : Outport
  C : Outport  Port=2
  wires:
  Half Adder1/1(Sum) -> S/1
  Half Adder/1(Sum) -> Half Adder1/1(A)
  Half Adder/2(Carry) -> OR/2
  X/1 -> Half Adder/1(A)
  Z/1 -> Half Adder1/2(B)
  OR/1 -> C/1
  Y/1 -> Half Adder/2(B)
  Half Adder1/2(Carry) -> OR/1

== system Multiplier/8-bit_Multiplier/Multiplier/Multiplier Building Block55/Full Adder ==
  X : Inport
  Y : Inport  Port=2
  Z : Inport  Port=3
  Half Adder : Subsystem
  Half Adder1 : Subsystem
  OR : Logic  Operator=OR  IconShape=distinctive  AllPortsSameDT=off  OutDataTypeStr=boolean
  S : Outport
  C : Outport  Port=2
  wires:
  Half Adder1/1(Sum) -> S/1
  Half Adder/1(Sum) -> Half Adder1/1(A)
  Half Adder/2(Carry) -> OR/2
  X/1 -> Half Adder/1(A)
  Z/1 -> Half Adder1/2(B)
  OR/1 -> C/1
  Y/1 -> Half Adder/2(B)
  Half Adder1/2(Carry) -> OR/1

== system Multiplier/8-bit_Multiplier/Multiplier/Multiplier Building Block56/Full Adder ==
  X : Inport
  Y : Inport  Port=2
  Z : Inport  Port=3
  Half Adder : Subsystem
  Half Adder1 : Subsystem
  OR : Logic  Operator=OR  IconShape=distinctive  AllPortsSameDT=off  OutDataTypeStr=boolean
  S : Outport
  C : Outport  Port=2
  wires:
  Half Adder1/1(Sum) -> S/1
  Half Adder/1(Sum) -> Half Adder1/1(A)
  Half Adder/2(Carry) -> OR/2
  X/1 -> Half Adder/1(A)
  Z/1 -> Half Adder1/2(B)
  OR/1 -> C/1
  Y/1 -> Half Adder/2(B)
  Half Adder1/2(Carry) -> OR/1

== system Multiplier/8-bit_Multiplier/Multiplier/Multiplier Building Block57/Full Adder ==
  X : Inport
  Y : Inport  Port=2
  Z : Inport  Port=3
  Half Adder : Subsystem
  Half Adder1 : Subsystem
  OR : Logic  Operator=OR  IconShape=distinctive  AllPortsSameDT=off  OutDataTypeStr=boolean
  S : Outport
  C : Outport  Port=2
  wires:
  Half Adder1/1(Sum) -> S/1
  Half Adder/1(Sum) -> Half Adder1/1(A)
  Half Adder/2(Carry) -> OR/2
  X/1 -> Half Adder/1(A)
  Z/1 -> Half Adder1/2(B)
  OR/1 -> C/1
  Y/1 -> Half Adder/2(B)
  Half Adder1/2(Carry) -> OR/1

== system Multiplier/8-bit_Multiplier/Multiplier/Multiplier Building Block58/Full Adder ==
  X : Inport
  Y : Inport  Port=2
  Z : Inport  Port=3
  Half Adder : Subsystem
  Half Adder1 : Subsystem
  OR : Logic  Operator=OR  IconShape=distinctive  AllPortsSameDT=off  OutDataTypeStr=boolean
  S : Outport
  C : Outport  Port=2
  wires:
  Half Adder1/1(Sum) -> S/1
  Half Adder/1(Sum) -> Half Adder1/1(A)
  Half Adder/2(Carry) -> OR/2
  X/1 -> Half Adder/1(A)
  Z/1 -> Half Adder1/2(B)
  OR/1 -> C/1
  Y/1 -> Half Adder/2(B)
  Half Adder1/2(Carry) -> OR/1

== system Multiplier/8-bit_Multiplier/Multiplier/Multiplier Building Block59/Full Adder ==
  X : Inport
  Y : Inport  Port=2
  Z : Inport  Port=3
  Half Adder : Subsystem
  Half Adder1 : Subsystem
  OR : Logic  Operator=OR  IconShape=distinctive  AllPortsSameDT=off  OutDataTypeStr=boolean
  S : Outport
  C : Outport  Port=2
  wires:
  Half Adder1/1(Sum) -> S/1
  Half Adder/1(Sum) -> Half Adder1/1(A)
  Half Adder/2(Carry) -> OR/2
  X/1 -> Half Adder/1(A)
  Z/1 -> Half Adder1/2(B)
  OR/1 -> C/1
  Y/1 -> Half Adder/2(B)
  Half Adder1/2(Carry) -> OR/1

== system Multiplier/8-bit_Multiplier/Multiplier/Multiplier Building Block6/Full Adder ==
  X : Inport
  Y : Inport  Port=2
  Z : Inport  Port=3
  Half Adder : Subsystem
  Half Adder1 : Subsystem
  OR : Logic  Operator=OR  IconShape=distinctive  AllPortsSameDT=off  OutDataTypeStr=boolean
  S : Outport
  C : Outport  Port=2
  wires:
  Half Adder1/1(Sum) -> S/1
  Half Adder/1(Sum) -> Half Adder1/1(A)
  Half Adder/2(Carry) -> OR/2
  X/1 -> Half Adder/1(A)
  Z/1 -> Half Adder1/2(B)
  OR/1 -> C/1
  Y/1 -> Half Adder/2(B)
  Half Adder1/2(Carry) -> OR/1

== system Multiplier/8-bit_Multiplier/Multiplier/Multiplier Building Block60/Full Adder ==
  X : Inport
  Y : Inport  Port=2
  Z : Inport  Port=3
  Half Adder : Subsystem
  Half Adder1 : Subsystem
  OR : Logic  Operator=OR  IconShape=distinctive  AllPortsSameDT=off  OutDataTypeStr=boolean
  S : Outport
  C : Outport  Port=2
  wires:
  Half Adder1/1(Sum) -> S/1
  Half Adder/1(Sum) -> Half Adder1/1(A)
  Half Adder/2(Carry) -> OR/2
  X/1 -> Half Adder/1(A)
  Z/1 -> Half Adder1/2(B)
  OR/1 -> C/1
  Y/1 -> Half Adder/2(B)
  Half Adder1/2(Carry) -> OR/1

== system Multiplier/8-bit_Multiplier/Multiplier/Multiplier Building Block61/Full Adder ==
  X : Inport
  Y : Inport  Port=2
  Z : Inport  Port=3
  Half Adder : Subsystem
  Half Adder1 : Subsystem
  OR : Logic  Operator=OR  IconShape=distinctive  AllPortsSameDT=off  OutDataTypeStr=boolean
  S : Outport
  C : Outport  Port=2
  wires:
  Half Adder1/1(Sum) -> S/1
  Half Adder/1(Sum) -> Half Adder1/1(A)
  Half Adder/2(Carry) -> OR/2
  X/1 -> Half Adder/1(A)
  Z/1 -> Half Adder1/2(B)
  OR/1 -> C/1
  Y/1 -> Half Adder/2(B)
  Half Adder1/2(Carry) -> OR/1

== system Multiplier/8-bit_Multiplier/Multiplier/Multiplier Building Block62/Full Adder ==
  X : Inport
  Y : Inport  Port=2
  Z : Inport  Port=3
  Half Adder : Subsystem
  Half Adder1 : Subsystem
  OR : Logic  Operator=OR  IconShape=distinctive  AllPortsSameDT=off  OutDataTypeStr=boolean
  S : Outport
  C : Outport  Port=2
  wires:
  Half Adder1/1(Sum) -> S/1
  Half Adder/1(Sum) -> Half Adder1/1(A)
  Half Adder/2(Carry) -> OR/2
  X/1 -> Half Adder/1(A)
  Z/1 -> Half Adder1/2(B)
  OR/1 -> C/1
  Y/1 -> Half Adder/2(B)
  Half Adder1/2(Carry) -> OR/1

== system Multiplier/8-bit_Multiplier/Multiplier/Multiplier Building Block63/Full Adder ==
  X : Inport
  Y : Inport  Port=2
  Z : Inport  Port=3
  Half Adder : Subsystem
  Half Adder1 : Subsystem
  OR : Logic  Operator=OR  IconShape=distinctive  AllPortsSameDT=off  OutDataTypeStr=boolean
  S : Outport
  C : Outport  Port=2
  wires:
  Half Adder1/1(Sum) -> S/1
  Half Adder/1(Sum) -> Half Adder1/1(A)
  Half Adder/2(Carry) -> OR/2
  X/1 -> Half Adder/1(A)
  Z/1 -> Half Adder1/2(B)
  OR/1 -> C/1
  Y/1 -> Half Adder/2(B)
  Half Adder1/2(Carry) -> OR/1

== system Multiplier/8-bit_Multiplier/Multiplier/Multiplier Building Block7/Full Adder ==
  X : Inport
  Y : Inport  Port=2
  Z : Inport  Port=3
  Half Adder : Subsystem
  Half Adder1 : Subsystem
  OR : Logic  Operator=OR  IconShape=distinctive  AllPortsSameDT=off  OutDataTypeStr=boolean
  S : Outport
  C : Outport  Port=2
  wires:
  Half Adder1/1(Sum) -> S/1
  Half Adder/1(Sum) -> Half Adder1/1(A)
  Half Adder/2(Carry) -> OR/2
  X/1 -> Half Adder/1(A)
  Z/1 -> Half Adder1/2(B)
  OR/1 -> C/1
  Y/1 -> Half Adder/2(B)
  Half Adder1/2(Carry) -> OR/1

== system Multiplier/8-bit_Multiplier/Multiplier/Multiplier Building Block8/Full Adder ==
  X : Inport
  Y : Inport  Port=2
  Z : Inport  Port=3
  Half Adder : Subsystem
  Half Adder1 : Subsystem
  OR : Logic  Operator=OR  IconShape=distinctive  AllPortsSameDT=off  OutDataTypeStr=boolean
  S : Outport
  C : Outport  Port=2
  wires:
  Half Adder1/1(Sum) -> S/1
  Half Adder/1(Sum) -> Half Adder1/1(A)
  Half Adder/2(Carry) -> OR/2
  X/1 -> Half Adder/1(A)
  Z/1 -> Half Adder1/2(B)
  OR/1 -> C/1
  Y/1 -> Half Adder/2(B)
  Half Adder1/2(Carry) -> OR/1

== system Multiplier/8-bit_Multiplier/Multiplier/Multiplier Building Block9/Full Adder ==
  X : Inport
  Y : Inport  Port=2
  Z : Inport  Port=3
  Half Adder : Subsystem
  Half Adder1 : Subsystem
  OR : Logic  Operator=OR  IconShape=distinctive  AllPortsSameDT=off  OutDataTypeStr=boolean
  S : Outport
  C : Outport  Port=2
  wires:
  Half Adder1/1(Sum) -> S/1
  Half Adder/1(Sum) -> Half Adder1/1(A)
  Half Adder/2(Carry) -> OR/2
  X/1 -> Half Adder/1(A)
  Z/1 -> Half Adder1/2(B)
  OR/1 -> C/1
  Y/1 -> Half Adder/2(B)
  Half Adder1/2(Carry) -> OR/1

== system Multiplier/8-bit_Multiplier/Multiplier/Multiplier Building Block/Full Adder/Half Adder ==
  A : Inport
  B : Inport  Port=2
  AND : Logic  IconShape=distinctive  AllPortsSameDT=off  OutDataTypeStr=boolean
  XOR : Logic  Operator=XOR  IconShape=distinctive  AllPortsSameDT=off  OutDataTypeStr=boolean
  Sum : Outport
  Carry : Outport  Port=2
  wires:
  AND/1 -> Carry/1
  XOR/1 -> Sum/1
  B/1 -> XOR/2, AND/2
  A/1 -> AND/1, XOR/1

== system Multiplier/8-bit_Multiplier/Multiplier/Multiplier Building Block/Full Adder/Half Adder1 ==
  A : Inport
  B : Inport  Port=2
  AND : Logic  IconShape=distinctive  AllPortsSameDT=off  OutDataTypeStr=boolean
  XOR : Logic  Operator=XOR  IconShape=distinctive  AllPortsSameDT=off  OutDataTypeStr=boolean
  Sum : Outport
  Carry : Outport  Port=2
  wires:
  AND/1 -> Carry/1
  XOR/1 -> Sum/1
  B/1 -> XOR/2, AND/2
  A/1 -> AND/1, XOR/1

== system Multiplier/8-bit_Multiplier/Multiplier/Multiplier Building Block1/Full Adder/Half Adder ==
  A : Inport
  B : Inport  Port=2
  AND : Logic  IconShape=distinctive  AllPortsSameDT=off  OutDataTypeStr=boolean
  XOR : Logic  Operator=XOR  IconShape=distinctive  AllPortsSameDT=off  OutDataTypeStr=boolean
  Sum : Outport
  Carry : Outport  Port=2
  wires:
  AND/1 -> Carry/1
  XOR/1 -> Sum/1
  B/1 -> XOR/2, AND/2
  A/1 -> AND/1, XOR/1

== system Multiplier/8-bit_Multiplier/Multiplier/Multiplier Building Block1/Full Adder/Half Adder1 ==
  A : Inport
  B : Inport  Port=2
  AND : Logic  IconShape=distinctive  AllPortsSameDT=off  OutDataTypeStr=boolean
  XOR : Logic  Operator=XOR  IconShape=distinctive  AllPortsSameDT=off  OutDataTypeStr=boolean
  Sum : Outport
  Carry : Outport  Port=2
  wires:
  AND/1 -> Carry/1
  XOR/1 -> Sum/1
  B/1 -> XOR/2, AND/2
  A/1 -> AND/1, XOR/1

== system Multiplier/8-bit_Multiplier/Multiplier/Multiplier Building Block10/Full Adder/Half Adder ==
  A : Inport
  B : Inport  Port=2
  AND : Logic  IconShape=distinctive  AllPortsSameDT=off  OutDataTypeStr=boolean
  XOR : Logic  Operator=XOR  IconShape=distinctive  AllPortsSameDT=off  OutDataTypeStr=boolean
  Sum : Outport
  Carry : Outport  Port=2
  wires:
  AND/1 -> Carry/1
  XOR/1 -> Sum/1
  B/1 -> XOR/2, AND/2
  A/1 -> AND/1, XOR/1

== system Multiplier/8-bit_Multiplier/Multiplier/Multiplier Building Block10/Full Adder/Half Adder1 ==
  A : Inport
  B : Inport  Port=2
  AND : Logic  IconShape=distinctive  AllPortsSameDT=off  OutDataTypeStr=boolean
  XOR : Logic  Operator=XOR  IconShape=distinctive  AllPortsSameDT=off  OutDataTypeStr=boolean
  Sum : Outport
  Carry : Outport  Port=2
  wires:
  AND/1 -> Carry/1
  XOR/1 -> Sum/1
  B/1 -> XOR/2, AND/2
  A/1 -> AND/1, XOR/1

== system Multiplier/8-bit_Multiplier/Multiplier/Multiplier Building Block11/Full Adder/Half Adder ==
  A : Inport
  B : Inport  Port=2
  AND : Logic  IconShape=distinctive  AllPortsSameDT=off  OutDataTypeStr=boolean
  XOR : Logic  Operator=XOR  IconShape=distinctive  AllPortsSameDT=off  OutDataTypeStr=boolean
  Sum : Outport
  Carry : Outport  Port=2
  wires:
  AND/1 -> Carry/1
  XOR/1 -> Sum/1
  B/1 -> XOR/2, AND/2
  A/1 -> AND/1, XOR/1

== system Multiplier/8-bit_Multiplier/Multiplier/Multiplier Building Block11/Full Adder/Half Adder1 ==
  A : Inport
  B : Inport  Port=2
  AND : Logic  IconShape=distinctive  AllPortsSameDT=off  OutDataTypeStr=boolean
  XOR : Logic  Operator=XOR  IconShape=distinctive  AllPortsSameDT=off  OutDataTypeStr=boolean
  Sum : Outport
  Carry : Outport  Port=2
  wires:
  AND/1 -> Carry/1
  XOR/1 -> Sum/1
  B/1 -> XOR/2, AND/2
  A/1 -> AND/1, XOR/1

== system Multiplier/8-bit_Multiplier/Multiplier/Multiplier Building Block12/Full Adder/Half Adder ==
  A : Inport
  B : Inport  Port=2
  AND : Logic  IconShape=distinctive  AllPortsSameDT=off  OutDataTypeStr=boolean
  XOR : Logic  Operator=XOR  IconShape=distinctive  AllPortsSameDT=off  OutDataTypeStr=boolean
  Sum : Outport
  Carry : Outport  Port=2
  wires:
  AND/1 -> Carry/1
  XOR/1 -> Sum/1
  B/1 -> XOR/2, AND/2
  A/1 -> AND/1, XOR/1

== system Multiplier/8-bit_Multiplier/Multiplier/Multiplier Building Block12/Full Adder/Half Adder1 ==
  A : Inport
  B : Inport  Port=2
  AND : Logic  IconShape=distinctive  AllPortsSameDT=off  OutDataTypeStr=boolean
  XOR : Logic  Operator=XOR  IconShape=distinctive  AllPortsSameDT=off  OutDataTypeStr=boolean
  Sum : Outport
  Carry : Outport  Port=2
  wires:
  AND/1 -> Carry/1
  XOR/1 -> Sum/1
  B/1 -> XOR/2, AND/2
  A/1 -> AND/1, XOR/1

== system Multiplier/8-bit_Multiplier/Multiplier/Multiplier Building Block13/Full Adder/Half Adder ==
  A : Inport
  B : Inport  Port=2
  AND : Logic  IconShape=distinctive  AllPortsSameDT=off  OutDataTypeStr=boolean
  XOR : Logic  Operator=XOR  IconShape=distinctive  AllPortsSameDT=off  OutDataTypeStr=boolean
  Sum : Outport
  Carry : Outport  Port=2
  wires:
  AND/1 -> Carry/1
  XOR/1 -> Sum/1
  B/1 -> XOR/2, AND/2
  A/1 -> AND/1, XOR/1

== system Multiplier/8-bit_Multiplier/Multiplier/Multiplier Building Block13/Full Adder/Half Adder1 ==
  A : Inport
  B : Inport  Port=2
  AND : Logic  IconShape=distinctive  AllPortsSameDT=off  OutDataTypeStr=boolean
  XOR : Logic  Operator=XOR  IconShape=distinctive  AllPortsSameDT=off  OutDataTypeStr=boolean
  Sum : Outport
  Carry : Outport  Port=2
  wires:
  AND/1 -> Carry/1
  XOR/1 -> Sum/1
  B/1 -> XOR/2, AND/2
  A/1 -> AND/1, XOR/1

== system Multiplier/8-bit_Multiplier/Multiplier/Multiplier Building Block14/Full Adder/Half Adder ==
  A : Inport
  B : Inport  Port=2
  AND : Logic  IconShape=distinctive  AllPortsSameDT=off  OutDataTypeStr=boolean
  XOR : Logic  Operator=XOR  IconShape=distinctive  AllPortsSameDT=off  OutDataTypeStr=boolean
  Sum : Outport
  Carry : Outport  Port=2
  wires:
  AND/1 -> Carry/1
  XOR/1 -> Sum/1
  B/1 -> XOR/2, AND/2
  A/1 -> AND/1, XOR/1

== system Multiplier/8-bit_Multiplier/Multiplier/Multiplier Building Block14/Full Adder/Half Adder1 ==
  A : Inport
  B : Inport  Port=2
  AND : Logic  IconShape=distinctive  AllPortsSameDT=off  OutDataTypeStr=boolean
  XOR : Logic  Operator=XOR  IconShape=distinctive  AllPortsSameDT=off  OutDataTypeStr=boolean
  Sum : Outport
  Carry : Outport  Port=2
  wires:
  AND/1 -> Carry/1
  XOR/1 -> Sum/1
  B/1 -> XOR/2, AND/2
  A/1 -> AND/1, XOR/1

== system Multiplier/8-bit_Multiplier/Multiplier/Multiplier Building Block15/Full Adder/Half Adder ==
  A : Inport
  B : Inport  Port=2
  AND : Logic  IconShape=distinctive  AllPortsSameDT=off  OutDataTypeStr=boolean
  XOR : Logic  Operator=XOR  IconShape=distinctive  AllPortsSameDT=off  OutDataTypeStr=boolean
  Sum : Outport
  Carry : Outport  Port=2
  wires:
  AND/1 -> Carry/1
  XOR/1 -> Sum/1
  B/1 -> XOR/2, AND/2
  A/1 -> AND/1, XOR/1

== system Multiplier/8-bit_Multiplier/Multiplier/Multiplier Building Block15/Full Adder/Half Adder1 ==
  A : Inport
  B : Inport  Port=2
  AND : Logic  IconShape=distinctive  AllPortsSameDT=off  OutDataTypeStr=boolean
  XOR : Logic  Operator=XOR  IconShape=distinctive  AllPortsSameDT=off  OutDataTypeStr=boolean
  Sum : Outport
  Carry : Outport  Port=2
  wires:
  AND/1 -> Carry/1
  XOR/1 -> Sum/1
  B/1 -> XOR/2, AND/2
  A/1 -> AND/1, XOR/1
